simulink model "nonlinear_system_with_C_theta"  (R2022b)
settings: Solver=VariableStepAuto  StartTime=0.0  StopTime=50  RelTol=1e-3
values from neighbouring files (symbols this model uses):
  c = 0.000477768    [lab05.m]
  f = 0.0088    [lab05.m]
  g = 9.807    [lab05.m]
  J = 0.0057    [lab05.m]
  Kb = 24.2e-3*60/(2*pi)    (= 0.231092977369)    [lab05.m]
  Km = 24.2*0.001    (= 0.0242)    [lab05.m]
  Ku = 12    [lab05.m]
  L = Pau*C_theta    [lab05.m]
  M = 51e-3    (= 0.051)    [lab05.m]
  Nr = 4.5    [lab05.m]
  r = 0.287727    [lab05.m]
  Ra = 2.21    [lab05.m]
libraries: cstblocks x2
settings Model: Creator=X1  LastModifiedBy=X1

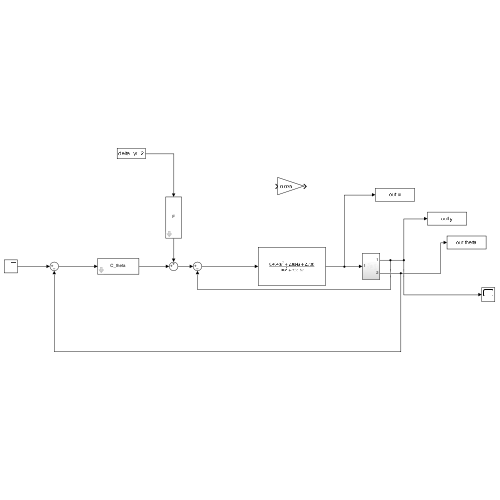
[thumbnail: Simulink's stored preview of the top-level diagram]
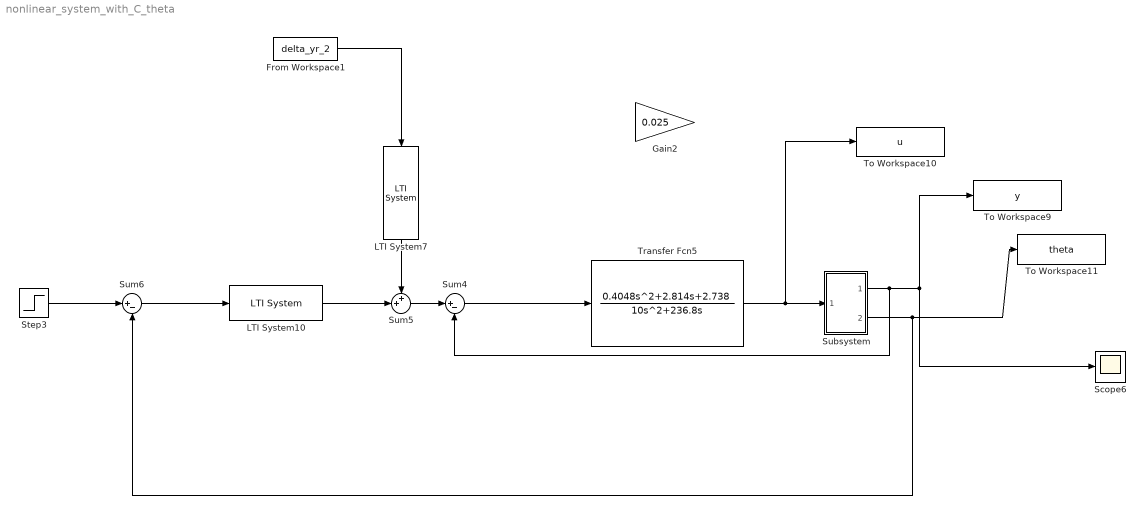
== system nonlinear_system_with_C_theta ==
  From Workspace1 : FromWorkspace  VariableName=delta_yr_2
  Gain2 : Gain  Gain=0.025
  LTI System10 : cstblocks/LTI System  sys=C_theta  IC=[]
  LTI System7 : cstblocks/LTI System  sys=F  IC=[]
  Scope6 : Scope
  Step3 : Step  Time=0  After=0  SampleTime=0
  Subsystem : Subsystem
  Sum4 : Sum  Inputs=|+-
  Sum5 : Sum  Inputs=++|
  Sum6 : Sum  Inputs=|+-
  To Workspace10 : ToWorkspace  VariableName=u  SaveFormat=Timeseries  SampleTime=-1
  To Workspace11 : ToWorkspace  VariableName=theta  SaveFormat=Timeseries  SampleTime=-1
  To Workspace9 : ToWorkspace  VariableName=y  SaveFormat=Structure With Time  SampleTime=-1
  Transfer Fcn5 : TransferFcn  Numerator=[0.4048 2.814 2.738]  Denominator=[10 236.8 0]
  wires:
  Transfer Fcn5/1 -> Subsystem/1(In1), To Workspace10/1
  Step3/1 -> Sum6/1
  Sum4/1 -> Transfer Fcn5/1
  LTI System10/1 -> Sum5/2
  LTI System7/1 -> Sum5/1
  Sum6/1 -> LTI System10/1
  From Workspace1/1 -> LTI System7/1
  Subsystem/2(Out2) -> To Workspace11/1, Sum6/2
  Sum5/1 -> Sum4/1
  Subsystem/1(Out1) -> To Workspace9/1, Scope6/1, Sum4/2

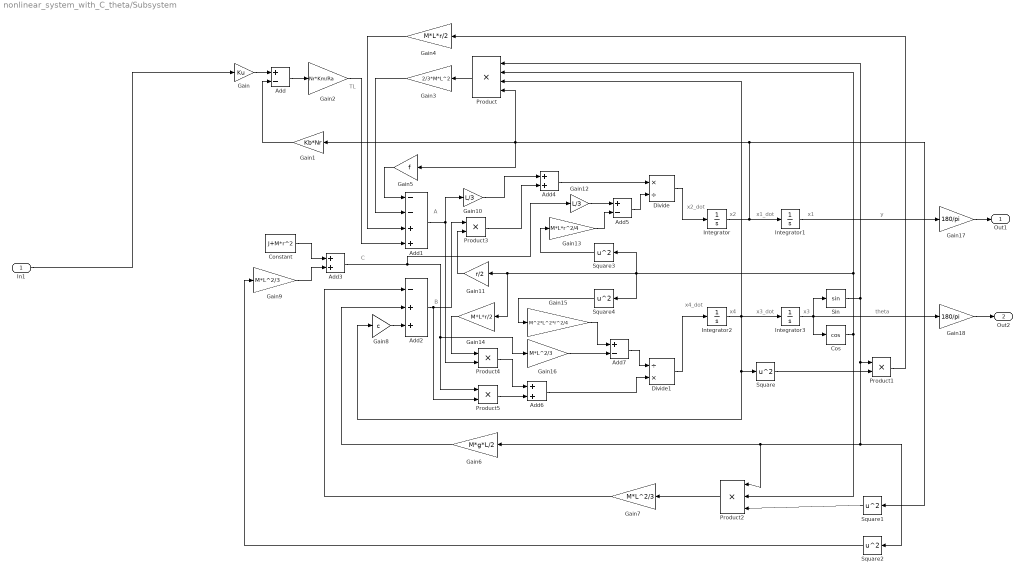
== system nonlinear_system_with_C_theta/Subsystem ==
  note: theta
  note: y
  note: x1
  note: x4_dot
  note: x2_dot
  note: C
  note: B
  note: A
  note: TL
  note: x3
  note: x3_dot
  note: x4
  note: x1_dot
  note: x2
  In1 : Inport
  Add : Sum  Inputs=+-
  Add1 : Sum  Inputs=--++
  Add2 : Sum  Inputs=-++
  Add3 : Sum
  Add4 : Sum
  Add5 : Sum  Inputs=+-
  Add6 : Sum
  Add7 : Sum  Inputs=+-
  Constant : Constant  Value=J+M*r^2
  Cos : Trigonometry  Operator=cos
  Divide : Product  Inputs=*/
  Divide1 : Product  Inputs=/*
  Gain : Gain  Gain=Ku
  Gain1 : Gain  Gain=Kb*Nr
  Gain10 : Gain  Gain=L/3
  Gain11 : Gain  Gain=r/2
  Gain12 : Gain  Gain=L/3
  Gain13 : Gain  Gain=M*L*r^2/4
  Gain14 : Gain  Gain=M*L*r/2
  Gain15 : Gain  Gain=M^2*L^2*r^2/4
  Gain16 : Gain  Gain=M*L^2/3
  Gain17 : Gain  Gain=180/pi
  Gain18 : Gain  Gain=180/pi
  Gain2 : Gain  Gain=Nr*Km/Ra
  Gain3 : Gain  Gain=2/3*M*L^2
  Gain4 : Gain  Gain=M*L*r/2
  Gain5 : Gain  Gain=f
  Gain6 : Gain  Gain=M*g*L/2
  Gain7 : Gain  Gain=M*L^2/3
  Gain8 : Gain  Gain=c
  Gain9 : Gain  Gain=M*L^2/3
  Integrator{,1..3} (4 alike) : Integrator
  Product : Product  Inputs=4
  Product{1,3..5} (4 alike) : Product
  Product2 : Product  Inputs=3
  Sin : Trigonometry
  Square{,1..4} (5 alike) : Math  Operator=square
  Out1 : Outport
  Out2 : Outport  Port=2
  wires:
  Cos/1 -> Product2/2, Product/2, Square4/1, Square3/1, Gain11/1, Gain14/1
  Integrator/1 -> Square1/1, Gain1/1, Gain5/1, Product/4, Integrator1/1
  Constant/1 -> Add3/1
  Integrator2/1 -> Product/3, Integrator3/1, Square/1, Gain8/1
  Add5/1 -> Divide/2
  Add3/1 -> Gain12/1, Gain16/1, Product5/1
  Gain7/1 -> Add2/1
  Add2/1 -> Product5/2, Product3/1
  Gain16/1 -> Add7/2
  Add1/1 -> Product4/2, Gain10/1
  Integrator3/1 -> Cos/1, Gain18/1, Sin/1
  Gain18/1 -> Out2/1
  Gain2/1 -> Add1/4
  Gain5/1 -> Add1/1
  Product2/1 -> Gain7/1
  In1/1 -> Gain/1
  Product1/1 -> Gain4/1
  Gain3/1 -> Add1/2
  Integrator1/1 -> Gain17/1
  Gain6/1 -> Add2/2
  Add4/1 -> Divide/1
  Sin/1 -> Product2/1, Gain6/1, Square2/1, Product1/1, Product/1
  Add7/1 -> Divide1/1
  Add/1 -> Gain2/1
  Square1/1 -> Product2/3
  Product3/1 -> Add4/2
  Product/1 -> Gain3/1
  Square/1 -> Product1/2
  Gain13/1 -> Add5/2
  Square2/1 -> Gain9/1
  Gain8/1 -> Add2/3
  Product5/1 -> Add6/2
  Product4/1 -> Add6/1
  Gain/1 -> Add/1
  Gain14/1 -> Product4/1
  Gain1/1 -> Add/2
  Gain4/1 -> Add1/3
  Gain9/1 -> Add3/2
  Divide/1 -> Integrator/1
  Square3/1 -> Gain13/1
  Square4/1 -> Gain15/1
  Gain11/1 -> Product3/2
  Add6/1 -> Divide1/2
  Divide1/1 -> Integrator2/1
  Gain15/1 -> Add7/1
  Gain10/1 -> Add4/1
  Gain12/1 -> Add5/1
  Gain17/1 -> Out1/1
